simulink model "ass3_2024a"  (R2024a)
settings: Solver=FixedStepAuto  StartTime=0.0  StopTime=inf  FixedStep=0.1  RelTol=1e-3
model workspace (MAT data in the model file):
  SL_ROS_VariableLengthArrays_MaxSizes.CommonInfo.ArrayTruncateAction = 'EmitWarning'
  SL_ROS_VariableLengthArrays_MaxSizes.MsgTypeMap = containers.Map
  SL_ROS_VariableLengthArrays_MaxSizes.MsgTypeMap.serialization.keys = {'sensor_msgs/Image'}
  SL_ROS_VariableLengthArrays_MaxSizes.MsgTypeMap.serialization.values{1}(1).PropertyName = 'Data'
  SL_ROS_VariableLengthArrays_MaxSizes.MsgTypeMap.serialization.values{1}(1).DataType = 'uint8'
  SL_ROS_VariableLengthArrays_MaxSizes.MsgTypeMap.serialization.values{1}(1).MaxLength = 921600
  SL_ROS_VariableLengthArrays_MaxSizes.MsgTypeMap.serialization.values{1}(2).PropertyName = 'Encoding'
  SL_ROS_VariableLengthArrays_MaxSizes.MsgTypeMap.serialization.values{1}(2).DataType = 'uint8'
  SL_ROS_VariableLengthArrays_MaxSizes.MsgTypeMap.serialization.values{1}(2).MaxLength = 128
  SL_ROS_VariableLengthArrays_MaxSizes.MsgTypeMap.serialization.uniformity = 0
  SL_ROS_VariableLengthArrays_MaxSizes.MsgTypeMap.serialization.keyType = 'char'
  SL_ROS_VariableLengthArrays_MaxSizes.MsgTypeMap.serialization.valueType = 'any'
undefined symbols (not defined in the file or in its folder): Angular, Linear, Rec, SDTV
libraries: robotlib x5, simulink x2, visionstatistics x1, visionconversions x1
settings Model: Creator=alice
settings OptimizationCC: DefaultParameterBehavior=Inlined  EnhancedBackFolding=on  PassReuseOutputArgsAs=Individual arguments  ZeroExternalMemoryAtStartup=off  ZeroInternalMemoryAtStartup=off  MaxStackSize=64  OptimizeBlockOrder=speed  DifferentSizesBufferReuse=on  OptimizationCustomize=off  EfficientTunableParamExpr=on
settings DebuggingCC: ParameterTunabilityLossMsg=error
settings HardwareCC: ProdBitPerPointer=32  ProdBitPerSizeT=32  ProdBitPerPtrDiffT=32  ProdLargestAtomicFloat=None  ProdIntDivRoundTo=Undefined  ProdEndianess=Unspecified  ProdWordSize=32  ProdHWDeviceType=Generic->Unspecified (assume 32-bit Generic)  UseEmbeddedCoderFeatures=off
settings SFSimCC: MATLABDynamicMemAlloc=off
settings RTWCC: Description=Embedded Coder  SystemTargetFile=ert.tlc  HardwareBoard=Robot Operating System (ROS)  TLCOptions="-aInlineSetEventsForThisBaseRateFcn=TLC_FALSE -aSuppressMultiTaskScheduler=TLC_FALSE  -aRateBasedStepFcn=0"  TemplateMakefile=ert_default_tmf  Toolchain=Catkin  TargetLang=C++
settings CodeAppCC: ForceParamTrailComments=on  IgnoreCustomStorageClasses=off  OperatorAnnotations=on  SimulinkDataObjDesc=on  SFDataObjDesc=on  InsertBlockDesc=on
settings ERTTargetCC: SupportNonInlinedSFcns=on  InlinedParameterPlacement=NonHierarchical

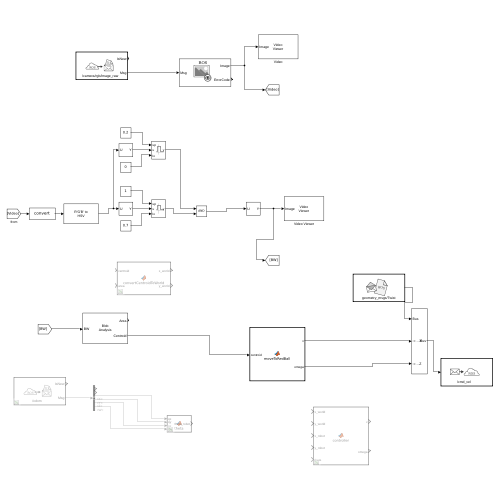
[thumbnail: Simulink's stored preview of the top-level diagram]
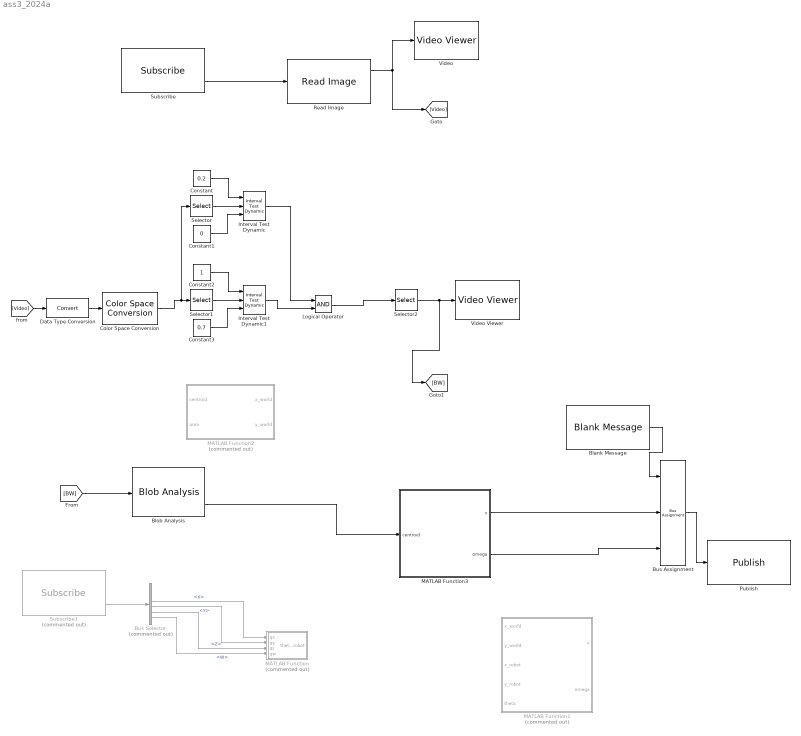
== system ass3_2024a ==
  Blank Message : robotlib/Blank Message  messageClass=Message  entityType=geometry_msgs/Twist  messageType=geometry_msgs/Twist  SampleTime=inf  legacyBusStruct=off
  Blob Analysis : visionstatistics/Blob Analysis  Tag=vipblks_row_conv  area=on  centroid=on  bBox=off  majorAxis=off  minorAxis=off  angle=off  eccentricity=off  equivDiameterSq=off  extent=off  perimeter=off  outDT=double  conn=8  isLabel=off  maxBlobs=2  warnIfNumBlobsExceeded=on  isCount=off  useMinArea=off  minArea=0  useMaxArea=off  maxArea=intmax('uint32')  excludeBorderBlob=off  isOutVarDim=off  isFill=on  fillValues=-1  roundingMode=Floor  overflowMode=off  prodOutputMode=Binary point scaling  prodOutputWordLength=32  prodOutputFracLength=16  accumMode=Binary point scaling  accumWordLength=32  accumFracLength=0  outputMode=Binary point scaling  outputWordLength=32  outputFracLength=16  firstCoeffMode=Binary point scaling  firstCoeffWordLength=16  firstCoeffFracLength=14  secondCoeffMode=Binary point scaling  secondCoeffWordLength=32  secondCoeffFracLength=16
  Bus Assignment : BusAssignment  AssignedSignals=Linear.X,Angular.Z
  Bus Selector : BusSelector  Commented=on  OutputSignals=Pose.Pose.Position.X,Pose.Pose.Position.Y,Pose.Pose.Orientation.X,Pose.Pose.Orientation.Y,Pose.Pose.Orientation.Z,Pose.Pose.Orientation.W
  Color Space Conversion : visionconversions/Color Space  Conversion  conversion=Obsolete  conversionActive=R'G'B' to HSV  wp_str=D65  rec=Rec. 601 (SDTV)  sys=1125/60/2:1  imagePorts=One multidimensional signal
  Constant : Constant  Value=0.2
  Constant1 : Constant  Value=0
  Constant2 : Constant
  Constant3 : Constant  Value=0.7
  Data Type Conversion : DataTypeConversion  SaturateOnIntegerOverflow=off  RndMeth=Floor
  Interval Test Dynamic : simulink/Logic and Bit Operations/Interval Test Dynamic  IntervalClosedRight=on  IntervalClosedLeft=on  OutDataTypeStr=boolean
  Interval Test Dynamic1 : simulink/Logic and Bit Operations/Interval Test Dynamic  IntervalClosedRight=on  IntervalClosedLeft=on  OutDataTypeStr=boolean
  Logical Operator : Logic  AllPortsSameDT=off  OutDataTypeStr=boolean
  MATLAB Function : MATLAB Function  Commented=on  TreatAsAtomicUnit=on
  MATLAB Function1 : MATLAB Function  Commented=on  TreatAsAtomicUnit=on
  MATLAB Function2 : MATLAB Function  Commented=on  TreatAsAtomicUnit=on
  MATLAB Function3 : MATLAB Function  TreatAsAtomicUnit=on
  Publish : robotlib/Publish  topicSource=Select from ROS network  topic=/cmd_vel  messageType=geometry_msgs/Twist  legacyBusStruct=off  messageQueueLength=1
  Read Image : robotlib/Read Image  MaximumImageSize=[480, 640]  ImageEncoding=rgb8  ShowAlphaOutput=off  ShowErrorCodeOutput=on  VariableSizeOutputs=off
  Selector : Selector  NumberOfDimensions=3  InputPortWidth=3  IndexOptions=Index vector (dialog),Index vector (dialog),Index vector (dialog)  Indices=[1:480],[1:640],1  OutputSizes=1,1,1
  Selector1 : Selector  NumberOfDimensions=3  InputPortWidth=3  IndexOptions=Index vector (dialog),Index vector (dialog),Index vector (dialog)  Indices=[1:480],[1:640],2  OutputSizes=1,1,1
  Selector2 : Selector  NumberOfDimensions=2  InputPortWidth=3  IndexOptions=Index vector (dialog),Index vector (dialog)  Indices=[1:480],[1:640]  OutputSizes=1,1
  Subscribe : robotlib/Subscribe  topicSource=Select from ROS network  topic=/camera/rgb/image_raw  messageType=sensor_msgs/Image  SampleTime=-1  legacyBusStruct=off  messageQueueLength=1
  Subscribe1 : robotlib/Subscribe  Commented=on  topicSource=Select from ROS network  topic=/odom  messageType=nav_msgs/Odometry  SampleTime=-1  legacyBusStruct=off  messageQueueLength=1
  Video : VideoViewer  FigPos=[78 933 1780 788]
  Video Viewer : VideoViewer  FigPos=[73 975 1856 788]
  wires:
  Subscribe/2 -> Read Image/1
  Read Image/1 -> [Video], Video/1
  Subscribe1/2 -> Bus Selector/1
  Bus Selector/3 -> MATLAB Function/1(qx)  "<X>"
  Bus Selector/4 -> MATLAB Function/2(qy)  "<Y>"
  Bus Selector/5 -> MATLAB Function/3(qz)  "<Z>"
  Bus Selector/6 -> MATLAB Function/4(qw)  "<W>"
  [Video] -> Data Type Conversion/1
  Data Type Conversion/1 -> Color Space Conversion/1
  Constant/1 -> Interval Test Dynamic/1
  Constant1/1 -> Interval Test Dynamic/3
  Selector/1 -> Interval Test Dynamic/2
  Selector1/1 -> Interval Test Dynamic1/2
  Constant3/1 -> Interval Test Dynamic1/3
  Constant2/1 -> Interval Test Dynamic1/1
  Color Space Conversion/1 -> Selector/1, Selector1/1
  [BW] -> Blob Analysis/1
  Interval Test Dynamic/1 -> Logical Operator/1
  Interval Test Dynamic1/1 -> Logical Operator/2
  Logical Operator/1 -> Selector2/1
  Selector2/1 -> [BW], Video Viewer/1
  Blank Message/1 -> Bus Assignment/1
  Bus Assignment/1 -> Publish/1
  Blob Analysis/2 -> MATLAB Function3/1(centroid)
  MATLAB Function3/1(v) -> Bus Assignment/2
  MATLAB Function3/2(omega) -> Bus Assignment/3

== matlab function ass3_2024a/MATLAB Function1 ==
  data: x_world input; y_world input; v output; x_robot input; y_robot input; theta input; omega output
function [v, omega] = controller(x_world, y_world,x_robot, y_robot, theta)
    % Estrai le coordinate del target dal vettore centroid
 
    
    % Parametri di guadagno proporzionale
    Kp = 0.5;         % Guadagno per la velocità lineare
    K_theta = 2.0;    % Guadagno per la velocità angolare

    % Calcolo dell'errore di posizione
    e_x = x_world - x_robot;
    e_y = y_world - y_robot;
    
    % Calcolo della distanza dal target
    distance = sqrt(e_x^2 + e_y^2);
    
    % Calcolo dell'angolo desiderato verso il target
    theta_desired = atan2(e_y, e_x);
    
    % Calcolo dell'errore angolare
    e_theta = theta_desired - theta;
    
    % Normalizzazione dell'errore angolare tra -pi e +pi
    e_theta = atan2(sin(e_theta), cos(e_theta));
    
    % Controllo proporzionale per la velocità lineare e angolare
    v = Kp * distance;
    omega = K_theta * e_theta;
    
    % Limita la velocità massima del robot (opzionale)
    v_max = 0.5;     % [m/s]
    omega_max = 1.0; % [rad/s]
    v = min(v, v_max);
    omega = min(max(omega, -omega_max), omega_max);
    
    % Ferma il robot se è molto vicino al target
    if distance < 0.1
        v = 0;
        omega = 0;
    end
end

== matlab function ass3_2024a/MATLAB Function ==
  data: qx input; theta_robot output; qy input; qz input; qw input
function theta_robot = theta(qx, qy, qz, qw)
    % Converti i quaternioni in angolo di eulero (yaw)
    % Formula per convertire quaternion a yaw:
    theta_robot = 2*atan2(qz,qw);
end

== matlab function ass3_2024a/MATLAB Function2 ==
  data: centroid input; x_world output; y_world output; area input
function [x_world, y_world] = convertCentroidToWorld(centroid,area)
   

% Estrai le coordinate del centroide
    x_centroid = centroid(1);
    y_centroid = centroid(2);
    
    % Funzione per convertire le coordinate del centroide da pixel a coordinate del mondo reale
    % x_centroid, y_centroid: coordinate del centroide in pixel
    % Z: distanza dell'oggetto dalla telecamera (in metri), fissa a 6 metri
    
    % Parametri della matrice di calibrazione K (inseriti direttamente nella funzione)
    f_x = 530.4669406576809;  % lunghezza focale in pixel (x)
    f_y = 530.4669406576809;  % lunghezza focale in pixel (y)
    c_x = 320.5;              % punto centrale in pixel (x)
    c_y = 240.5;              % punto centrale in pixel (y)
    
   d_p = 2 * sqrt(double(area(1,1)) / pi);

    Z = f_x*0.1/d_p; 
    
    % Calcolare le coordinate nel mondo reale
    x_world = (x_centroid - c_x) * Z / f_x;  % Coordinate reali X
    y_world = (y_centroid - c_y) * Z / f_y;  % Coordinate reali Y
end

== matlab function ass3_2024a/MATLAB Function3 ==
  data: centroid input; v output double; omega output double
function [v, omega] = moveToRedBall(centroid)
    % Parametri della telecamera
   
    x_img = 320.5;     % Centro dell'immagine in pixel (asse x)
    y_img = 240.5;     % Centro dell'immagine in pixel (asse y)


 % Estrai il centroide corretto dai dati
    x_sfera = double(centroid(1)); % Coordinata x del centroide
    y_sfera = double(centroid(2)); % Coordinata y del centroide
% CONTROLLOSFEREA - Calcola velocità lineare e angolare per raggiungere una sfera
%
% INPUT:
% x_sfera, y_sfera - coordinate del centroide della sfera
% x_img, y_img     - coordinate del centro dell'immagine
%
% OUTPUT:
% v                - velocità lineare
% omega            - velocità angolare

% Parametri del controllo
    K_ang = 0.005; % Guadagno proporzionale per la velocità angolare (ridotto)
    K_lin = 0.1;   % Guadagno proporzionale per la velocità lineare
    max_v = 0.5;   % Velocità lineare massima
    max_omega = 0.4; % Velocità angolare massima (ridotto)
    ang_tolerance = 0.05; % Soglia di tolleranza per l'errore angolare

    % Calcolo errore angolare
    e_ang = x_sfera - x_img;

    % Controllo proporzionale per velocità angolare
    if abs(e_ang) > ang_tolerance
        omega = K_ang * e_ang;
    else
        omega = 0; % Se l'errore è piccolo, non corregge
    end

    % Saturazione della velocità angolare
    omega = min(max(omega, -max_omega), max_omega);

    % Velocità lineare
    if abs(e_ang) < ang_tolerance
        % Se l'errore angolare è sotto la tolleranza, avanza dritto
        v = max_v;
    else
        % Altrimenti rallenta per riallinearsi
        v = K_lin;
    end

    % Saturazione della velocità lineare
    v = min(max(v, 0), max_v);

    % Fermo il robot se il centroide non è visibile
    if isnan(x_sfera) || isnan(y_sfera)
        v = 0;
        omega = 0;
    end
end
